simulink model "Position_Control_Closed_Loop"  (R2021b)
settings: Solver=ode3  StartTime=0.0  StopTime=20  FixedStep=ts  RelTol=1e-3  EnableMultiTasking=on
undefined symbols (not defined in the file or in its folder): ts
libraries: arduinolib x3, simulink x1, arduinosensorlib x1, dspsrcs4 x1
settings Model: ExtModeTrigDuration=2  Creator=tsuga  LastModifiedBy=karteek
settings SolverCC: AutoInsertRateTranBlk=on
settings DataIOCC: SaveOutput=off  SignalLogging=off  DSMLogging=off  SaveTime=off  ReturnWorkspaceOutputs=off
settings OptimizationCC: EnhancedBackFolding=on  PassReuseOutputArgsAs=Individual arguments  ZeroExternalMemoryAtStartup=off  ZeroInternalMemoryAtStartup=off  MaxStackSize=64  OptimizeBlockOrder=speed  DifferentSizesBufferReuse=on  OptimizationCustomize=off  EfficientTunableParamExpr=on
settings DebuggingCC: ParameterTunabilityLossMsg=error
settings HardwareCC: ProdBitPerInt=16  ProdBitPerPointer=16  ProdBitPerSizeT=16  ProdBitPerPtrDiffT=16  ProdLargestAtomicFloat=None  ProdWordSize=8  ProdHWDeviceType=Atmel->AVR
settings SFSimCC: MATLABDynamicMemAlloc=off
settings RTWCC: Description=Embedded Coder  SystemTargetFile=ert.tlc  HardwareBoard=Arduino Leonardo  TemplateMakefile=ert_default_tmf  Toolchain=Arduino AVR  BuildConfiguration=Faster Runs
settings CodeAppCC: ForceParamTrailComments=on  IgnoreCustomStorageClasses=off  OperatorAnnotations=on  SimulinkDataObjDesc=on  SFDataObjDesc=on  InsertBlockDesc=on
settings ERTTargetCC: SupportContinuousTime=on  SupportVariableSizeSignals=on  ExtModeTransport=5  ExtModeStaticAllocSize=250  ExtModeMexFile=ext_serial_win32_comm_leonardo

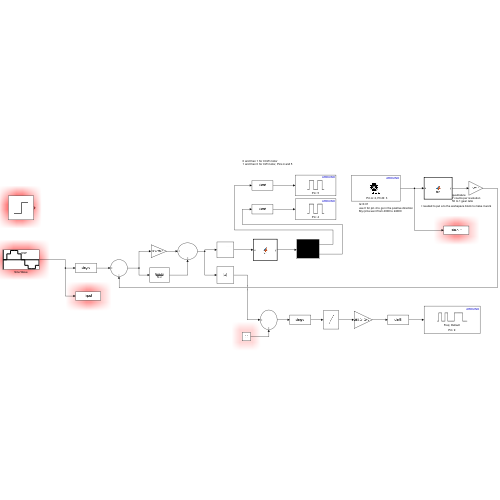
[thumbnail: Simulink's stored preview of the top-level diagram]
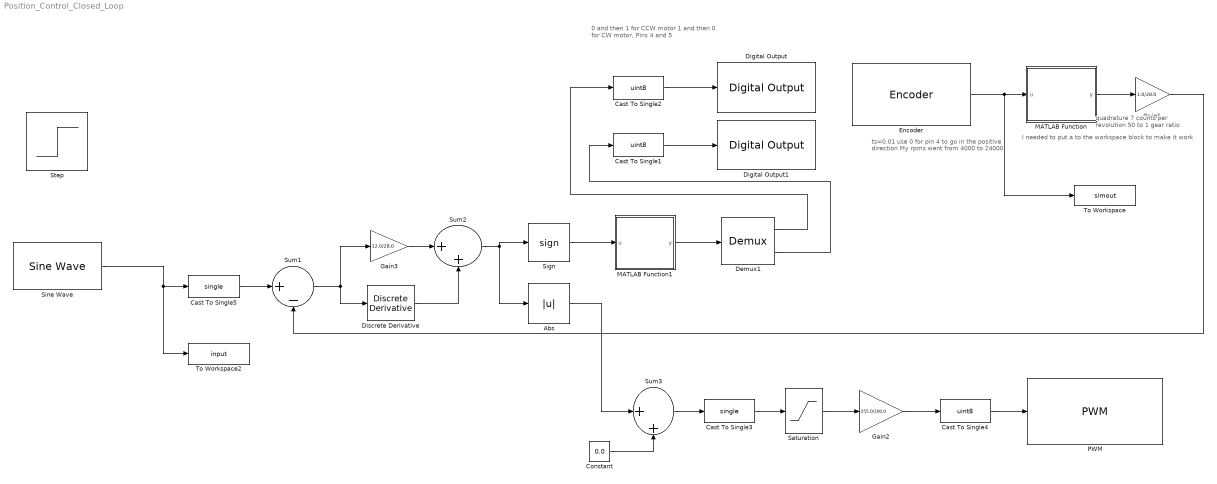
== system Position_Control_Closed_Loop ==
  note: quadrature
      | 7 counts per revolution
      | 50 to 1 gear ratio
  note: ts=0.01
      | use 0 for pin 4 to go in the positive direction
      | My rpms went from 4000 to 24000
  note: I needed to put a to the workspace block to make it work
  note: 0 and then 1 for CCW motor
      | 1 and then 0 for CW motor, Pins 4 and 5
  Abs : Abs
  Cast To Single1 : DataTypeConversion  OutDataTypeStr=uint8
  Cast To Single2 : DataTypeConversion  OutDataTypeStr=uint8
  Cast To Single3 : DataTypeConversion  OutDataTypeStr=single
  Cast To Single4 : DataTypeConversion  OutDataTypeStr=uint8
  Cast To Single5 : DataTypeConversion  OutDataTypeStr=single
  Constant : Constant  Value=0.0  SampleTime=ts
  Demux1 : Demux  Outputs=2
  Digital Output : arduinolib/Digital Output  pinNumber=5  Direction=output  blockPlatform=arduino
  Digital Output1 : arduinolib/Digital Output  pinNumber=4  Direction=output  blockPlatform=arduino
  Discrete Derivative : simulink/Discrete/Discrete Derivative  gainval=0.3  ICPrevScaledInput=0.0  OutMin=[]  OutMax=[]  OutDataType=fixdt(1, 16)  OutScaling=2^-10  DoSatur=off
  Encoder : arduinosensorlib/Encoder  InputA=2  InputB=3  Mode=No reset  SampleTime=ts
      settings: SourceProductBaseCode=ARDUINO
  Gain1 : Gain  Gain=1.0/28.0
  Gain2 : Gain  Gain=255.0/100.0
  Gain3 : Gain  Gain=12.0/28.0
  MATLAB Function : MATLAB Function  TreatAsAtomicUnit=on
  MATLAB Function1 : MATLAB Function  TreatAsAtomicUnit=on
  PWM : arduinolib/PWM  pinNumber=9  frequencyType=Default  desiredFrequency=490.2  achievableFrequency=490.2
  Saturation : Saturate  UpperLimit=100.0  LowerLimit=0.0
  Sign : Signum
  Sine Wave : dspsrcs4/Sine Wave  Amplitude=50  Frequency=0.2  Phase=0  SampleMode=Discrete  OutComplex=Real  CompMethod=Trigonometric fcn  TableSize=Speed  SampleTime=ts  SamplesPerFrame=1  ResetState=Restart at time zero  OutputFrames=off  dataType=double  wordLen=16  udDataType=sfix(16)  fracBitsMode=Best precision  numFracBits=15  OutDataTypeStr=double  LastOutDataTypeStr=double
  Step : Step  SampleTime=ts
  Sum1 : Sum  Inputs=|+-
  Sum2 : Sum  Inputs=|++
  Sum3 : Sum  Inputs=|++
  To Workspace : ToWorkspace  VariableName=simout  SampleTime=ts
      settings: Save2DSignal=2-D array (concatenate along first dimension)
  To Workspace2 : ToWorkspace  VariableName=input  SampleTime=ts
      settings: Save2DSignal=2-D array (concatenate along first dimension)
  wires:
  Cast To Single3/1 -> Saturation/1
  Saturation/1 -> Gain2/1
  Gain2/1 -> Cast To Single4/1
  Cast To Single4/1 -> PWM/1
  Cast To Single1/1 -> Digital Output1/1
  Cast To Single2/1 -> Digital Output/1
  Sum3/1 -> Cast To Single3/1
  Constant/1 -> Sum3/2
  Sine Wave/1 -> Cast To Single5/1, To Workspace2/1
  Encoder/1 -> MATLAB Function/1(u), To Workspace/1
  MATLAB Function/1(y) -> Gain1/1
  Gain1/1 -> Sum1/2
  Sum1/1 -> Gain3/1, Discrete Derivative/1
  Cast To Single5/1 -> Sum1/1
  Gain3/1 -> Sum2/1
  Discrete Derivative/1 -> Sum2/2
  Sum2/1 -> Sign/1, Abs/1
  Abs/1 -> Sum3/1
  Sign/1 -> MATLAB Function1/1(u)
  MATLAB Function1/1(y) -> Demux1/1
  Demux1/1 -> Cast To Single2/1
  Demux1/2 -> Cast To Single1/1

== matlab function Position_Control_Closed_Loop/MATLAB Function ==
  data: u input; y output
function y = fcn(u)
%#codegen

% xx = typecast(u,'single');
% y=xx(1);

y=single(u);  % this method worked

== matlab function Position_Control_Closed_Loop/MATLAB Function1 ==
  data: u input; y output
function y = fcn(u)


y = uint8(zeros(1,2));

if u >= 0
    y(1) = 0;
    y(2) = 1;

elseif u < 0
    y(1) = 1;
    y(2) = 0;

end
